simulink model "BouncingBallExample_Simulink"  (R2023a)
settings: Solver=FixedStepAuto  StartTime=0.0  StopTime=10  FixedStep=0.0001  RelTol=1e-3
libraries: simulink x1
settings Model: Creator=basti  LastModifiedBy=basti

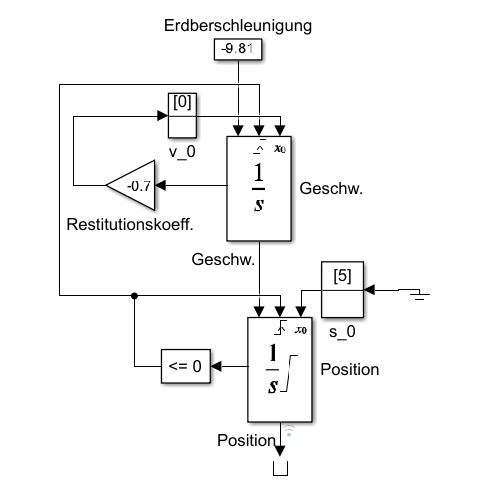
[thumbnail: Simulink's stored preview of the top-level diagram]
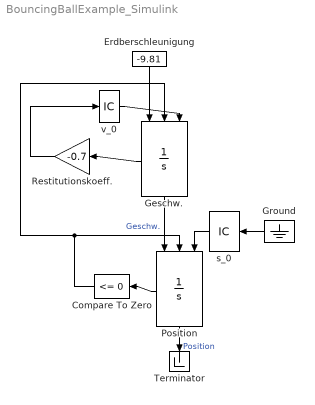
== system BouncingBallExample_Simulink ==
  Compare To Zero : simulink/Logic and Bit Operations/Compare To Zero  relop=<=  OutDataTypeStr=boolean
  Erdberschleunigung : Constant  Value=-9.81
  Geschw. : Integrator  ExternalReset=rising  InitialConditionSource=external  ShowStatePort=on
  Ground : Ground
  Position : Integrator  ExternalReset=rising  InitialConditionSource=external  LimitOutput=on  LowerSaturationLimit=0  ShowStatePort=on
  Restitutionskoeff. : Gain  Gain=-0.7  SaturateOnIntegerOverflow=on  OutDataTypeStr=Inherit: Same as input  ParamDataTypeStr=Inherit: Same as input
  Terminator : Terminator
  s_0 : InitialCondition  Value=5
  v_0 : InitialCondition  Value=0
  wires:
  Geschw./State -> Restitutionskoeff./1
  Position/1 -> Terminator/1  "Position"
  Position/State -> Compare To Zero/1
  Geschw./1 -> Position/1  "Geschw."
  Compare To Zero/1 -> Position/2, Geschw./2
  v_0/1 -> Geschw./3
  s_0/1 -> Position/3
  Restitutionskoeff./1 -> v_0/1
  Ground/1 -> s_0/1
  Erdberschleunigung/1 -> Geschw./1
